simulink model "project"  (R2018b)
settings: Solver=VariableStepAuto  StartTime=0.0  StopTime=10.0  RelTol=1e-3
libraries: commutil2 x4
(part 2 of 2)

== system project/mul_div/mul/4bitAdder0/FA2 ==
  In2 : Inport
  In3 : Inport  Port=2
  In4 : Inport  Port=3
  Logical Operator : Logic  Operator=XOR  IconShape=distinctive  AllPortsSameDT=off  OutDataTypeStr=boolean
  Logical Operator1 : Logic  Operator=XOR  IconShape=distinctive  AllPortsSameDT=off  OutDataTypeStr=boolean
  Logical Operator2 : Logic  IconShape=distinctive  AllPortsSameDT=off  OutDataTypeStr=boolean
  Logical Operator3 : Logic  IconShape=distinctive  AllPortsSameDT=off  OutDataTypeStr=boolean
  Logical Operator4 : Logic  Operator=OR  IconShape=distinctive  AllPortsSameDT=off  OutDataTypeStr=boolean
  Out2 : Outport
  Out1 : Outport  Port=2
  wires:
  Logical Operator2/1 -> Logical Operator4/1
  Logical Operator3/1 -> Logical Operator4/2
  Logical Operator1/1 -> Out2/1
  In4/1 -> Logical Operator2/2, Logical Operator1/2
  In3/1 -> Logical Operator3/2, Logical Operator/2
  In2/1 -> Logical Operator3/1, Logical Operator/1
  Logical Operator/1 -> Logical Operator1/1, Logical Operator2/1
  Logical Operator4/1 -> Out1/1

== system project/mul_div/mul/4bitAdder0/FA3 ==
  In2 : Inport
  In3 : Inport  Port=2
  In4 : Inport  Port=3
  Logical Operator : Logic  Operator=XOR  IconShape=distinctive  AllPortsSameDT=off  OutDataTypeStr=boolean
  Logical Operator1 : Logic  Operator=XOR  IconShape=distinctive  AllPortsSameDT=off  OutDataTypeStr=boolean
  Logical Operator2 : Logic  IconShape=distinctive  AllPortsSameDT=off  OutDataTypeStr=boolean
  Logical Operator3 : Logic  IconShape=distinctive  AllPortsSameDT=off  OutDataTypeStr=boolean
  Logical Operator4 : Logic  Operator=OR  IconShape=distinctive  AllPortsSameDT=off  OutDataTypeStr=boolean
  Out2 : Outport
  Out1 : Outport  Port=2
  wires:
  Logical Operator2/1 -> Logical Operator4/1
  Logical Operator3/1 -> Logical Operator4/2
  Logical Operator1/1 -> Out2/1
  In4/1 -> Logical Operator2/2, Logical Operator1/2
  In3/1 -> Logical Operator3/2, Logical Operator/2
  In2/1 -> Logical Operator3/1, Logical Operator/1
  Logical Operator/1 -> Logical Operator1/1, Logical Operator2/1
  Logical Operator4/1 -> Out1/1

== system project/mul_div/mul/4bitAdder1/FA0 ==
  In2 : Inport
  In3 : Inport  Port=2
  In4 : Inport  Port=3
  Logical Operator : Logic  Operator=XOR  IconShape=distinctive  AllPortsSameDT=off  OutDataTypeStr=boolean
  Logical Operator1 : Logic  Operator=XOR  IconShape=distinctive  AllPortsSameDT=off  OutDataTypeStr=boolean
  Logical Operator2 : Logic  IconShape=distinctive  AllPortsSameDT=off  OutDataTypeStr=boolean
  Logical Operator3 : Logic  IconShape=distinctive  AllPortsSameDT=off  OutDataTypeStr=boolean
  Logical Operator4 : Logic  Operator=OR  IconShape=distinctive  AllPortsSameDT=off  OutDataTypeStr=boolean
  Out2 : Outport
  Out1 : Outport  Port=2
  wires:
  Logical Operator2/1 -> Logical Operator4/1
  Logical Operator3/1 -> Logical Operator4/2
  Logical Operator1/1 -> Out2/1
  In4/1 -> Logical Operator2/2, Logical Operator1/2
  In3/1 -> Logical Operator3/2, Logical Operator/2
  In2/1 -> Logical Operator3/1, Logical Operator/1
  Logical Operator/1 -> Logical Operator1/1, Logical Operator2/1
  Logical Operator4/1 -> Out1/1

== system project/mul_div/mul/4bitAdder1/FA1 ==
  In2 : Inport
  In3 : Inport  Port=2
  In4 : Inport  Port=3
  Logical Operator : Logic  Operator=XOR  IconShape=distinctive  AllPortsSameDT=off  OutDataTypeStr=boolean
  Logical Operator1 : Logic  Operator=XOR  IconShape=distinctive  AllPortsSameDT=off  OutDataTypeStr=boolean
  Logical Operator2 : Logic  IconShape=distinctive  AllPortsSameDT=off  OutDataTypeStr=boolean
  Logical Operator3 : Logic  IconShape=distinctive  AllPortsSameDT=off  OutDataTypeStr=boolean
  Logical Operator4 : Logic  Operator=OR  IconShape=distinctive  AllPortsSameDT=off  OutDataTypeStr=boolean
  Out2 : Outport
  Out1 : Outport  Port=2
  wires:
  Logical Operator2/1 -> Logical Operator4/1
  Logical Operator3/1 -> Logical Operator4/2
  Logical Operator1/1 -> Out2/1
  In4/1 -> Logical Operator2/2, Logical Operator1/2
  In3/1 -> Logical Operator3/2, Logical Operator/2
  In2/1 -> Logical Operator3/1, Logical Operator/1
  Logical Operator/1 -> Logical Operator1/1, Logical Operator2/1
  Logical Operator4/1 -> Out1/1

== system project/mul_div/mul/4bitAdder1/FA2 ==
  In2 : Inport
  In3 : Inport  Port=2
  In4 : Inport  Port=3
  Logical Operator : Logic  Operator=XOR  IconShape=distinctive  AllPortsSameDT=off  OutDataTypeStr=boolean
  Logical Operator1 : Logic  Operator=XOR  IconShape=distinctive  AllPortsSameDT=off  OutDataTypeStr=boolean
  Logical Operator2 : Logic  IconShape=distinctive  AllPortsSameDT=off  OutDataTypeStr=boolean
  Logical Operator3 : Logic  IconShape=distinctive  AllPortsSameDT=off  OutDataTypeStr=boolean
  Logical Operator4 : Logic  Operator=OR  IconShape=distinctive  AllPortsSameDT=off  OutDataTypeStr=boolean
  Out2 : Outport
  Out1 : Outport  Port=2
  wires:
  Logical Operator2/1 -> Logical Operator4/1
  Logical Operator3/1 -> Logical Operator4/2
  Logical Operator1/1 -> Out2/1
  In4/1 -> Logical Operator2/2, Logical Operator1/2
  In3/1 -> Logical Operator3/2, Logical Operator/2
  In2/1 -> Logical Operator3/1, Logical Operator/1
  Logical Operator/1 -> Logical Operator1/1, Logical Operator2/1
  Logical Operator4/1 -> Out1/1

== system project/mul_div/mul/4bitAdder1/FA3 ==
  In2 : Inport
  In3 : Inport  Port=2
  In4 : Inport  Port=3
  Logical Operator : Logic  Operator=XOR  IconShape=distinctive  AllPortsSameDT=off  OutDataTypeStr=boolean
  Logical Operator1 : Logic  Operator=XOR  IconShape=distinctive  AllPortsSameDT=off  OutDataTypeStr=boolean
  Logical Operator2 : Logic  IconShape=distinctive  AllPortsSameDT=off  OutDataTypeStr=boolean
  Logical Operator3 : Logic  IconShape=distinctive  AllPortsSameDT=off  OutDataTypeStr=boolean
  Logical Operator4 : Logic  Operator=OR  IconShape=distinctive  AllPortsSameDT=off  OutDataTypeStr=boolean
  Out2 : Outport
  Out1 : Outport  Port=2
  wires:
  Logical Operator2/1 -> Logical Operator4/1
  Logical Operator3/1 -> Logical Operator4/2
  Logical Operator1/1 -> Out2/1
  In4/1 -> Logical Operator2/2, Logical Operator1/2
  In3/1 -> Logical Operator3/2, Logical Operator/2
  In2/1 -> Logical Operator3/1, Logical Operator/1
  Logical Operator/1 -> Logical Operator1/1, Logical Operator2/1
  Logical Operator4/1 -> Out1/1

== system project/mul_div/mul/4bitAdder2/FA0 ==
  In2 : Inport
  In3 : Inport  Port=2
  In4 : Inport  Port=3
  Logical Operator : Logic  Operator=XOR  IconShape=distinctive  AllPortsSameDT=off  OutDataTypeStr=boolean
  Logical Operator1 : Logic  Operator=XOR  IconShape=distinctive  AllPortsSameDT=off  OutDataTypeStr=boolean
  Logical Operator2 : Logic  IconShape=distinctive  AllPortsSameDT=off  OutDataTypeStr=boolean
  Logical Operator3 : Logic  IconShape=distinctive  AllPortsSameDT=off  OutDataTypeStr=boolean
  Logical Operator4 : Logic  Operator=OR  IconShape=distinctive  AllPortsSameDT=off  OutDataTypeStr=boolean
  Out2 : Outport
  Out1 : Outport  Port=2
  wires:
  Logical Operator2/1 -> Logical Operator4/1
  Logical Operator3/1 -> Logical Operator4/2
  Logical Operator1/1 -> Out2/1
  In4/1 -> Logical Operator2/2, Logical Operator1/2
  In3/1 -> Logical Operator3/2, Logical Operator/2
  In2/1 -> Logical Operator3/1, Logical Operator/1
  Logical Operator/1 -> Logical Operator1/1, Logical Operator2/1
  Logical Operator4/1 -> Out1/1

== system project/mul_div/mul/4bitAdder2/FA1 ==
  In2 : Inport
  In3 : Inport  Port=2
  In4 : Inport  Port=3
  Logical Operator : Logic  Operator=XOR  IconShape=distinctive  AllPortsSameDT=off  OutDataTypeStr=boolean
  Logical Operator1 : Logic  Operator=XOR  IconShape=distinctive  AllPortsSameDT=off  OutDataTypeStr=boolean
  Logical Operator2 : Logic  IconShape=distinctive  AllPortsSameDT=off  OutDataTypeStr=boolean
  Logical Operator3 : Logic  IconShape=distinctive  AllPortsSameDT=off  OutDataTypeStr=boolean
  Logical Operator4 : Logic  Operator=OR  IconShape=distinctive  AllPortsSameDT=off  OutDataTypeStr=boolean
  Out2 : Outport
  Out1 : Outport  Port=2
  wires:
  Logical Operator2/1 -> Logical Operator4/1
  Logical Operator3/1 -> Logical Operator4/2
  Logical Operator1/1 -> Out2/1
  In4/1 -> Logical Operator2/2, Logical Operator1/2
  In3/1 -> Logical Operator3/2, Logical Operator/2
  In2/1 -> Logical Operator3/1, Logical Operator/1
  Logical Operator/1 -> Logical Operator1/1, Logical Operator2/1
  Logical Operator4/1 -> Out1/1

== system project/mul_div/mul/4bitAdder2/FA2 ==
  In2 : Inport
  In3 : Inport  Port=2
  In4 : Inport  Port=3
  Logical Operator : Logic  Operator=XOR  IconShape=distinctive  AllPortsSameDT=off  OutDataTypeStr=boolean
  Logical Operator1 : Logic  Operator=XOR  IconShape=distinctive  AllPortsSameDT=off  OutDataTypeStr=boolean
  Logical Operator2 : Logic  IconShape=distinctive  AllPortsSameDT=off  OutDataTypeStr=boolean
  Logical Operator3 : Logic  IconShape=distinctive  AllPortsSameDT=off  OutDataTypeStr=boolean
  Logical Operator4 : Logic  Operator=OR  IconShape=distinctive  AllPortsSameDT=off  OutDataTypeStr=boolean
  Out2 : Outport
  Out1 : Outport  Port=2
  wires:
  Logical Operator2/1 -> Logical Operator4/1
  Logical Operator3/1 -> Logical Operator4/2
  Logical Operator1/1 -> Out2/1
  In4/1 -> Logical Operator2/2, Logical Operator1/2
  In3/1 -> Logical Operator3/2, Logical Operator/2
  In2/1 -> Logical Operator3/1, Logical Operator/1
  Logical Operator/1 -> Logical Operator1/1, Logical Operator2/1
  Logical Operator4/1 -> Out1/1

== system project/mul_div/mul/4bitAdder2/FA3 ==
  In2 : Inport
  In3 : Inport  Port=2
  In4 : Inport  Port=3
  Logical Operator : Logic  Operator=XOR  IconShape=distinctive  AllPortsSameDT=off  OutDataTypeStr=boolean
  Logical Operator1 : Logic  Operator=XOR  IconShape=distinctive  AllPortsSameDT=off  OutDataTypeStr=boolean
  Logical Operator2 : Logic  IconShape=distinctive  AllPortsSameDT=off  OutDataTypeStr=boolean
  Logical Operator3 : Logic  IconShape=distinctive  AllPortsSameDT=off  OutDataTypeStr=boolean
  Logical Operator4 : Logic  Operator=OR  IconShape=distinctive  AllPortsSameDT=off  OutDataTypeStr=boolean
  Out2 : Outport
  Out1 : Outport  Port=2
  wires:
  Logical Operator2/1 -> Logical Operator4/1
  Logical Operator3/1 -> Logical Operator4/2
  Logical Operator1/1 -> Out2/1
  In4/1 -> Logical Operator2/2, Logical Operator1/2
  In3/1 -> Logical Operator3/2, Logical Operator/2
  In2/1 -> Logical Operator3/1, Logical Operator/1
  Logical Operator/1 -> Logical Operator1/1, Logical Operator2/1
  Logical Operator4/1 -> Out1/1
